simulink model "smm_with_grf_tilting_2d"  (R2014b)
settings: Solver=FixedStepDiscrete  StartTime=0.0  StopTime=inf  FixedStep=sample_time  RelTol=1e-3
undefined symbols (not defined in the file or in its folder): A_kalman_fourbar_gear, A_kalman_transverse, A_kalman_vertical, A_lpf_dtau, A_lpf_leg_spring, alpha_apex, B1_lpf_dtau, B1_lpf_leg_spring, B2_lpf_dtau, B2_lpf_leg_spring, B_kalman_fourbar_gear, B_kalman_transverse, B_kalman_vertical, b_virtual, boom_mount_angle, c_energy, C_kalman_fourbar_gear, C_kalman_transverse, C_kalman_vertical, com_leg_motor, com_torso, contact_threshold, control_start_time, d_vertical_boom_com_offset, d_vertical_com, d_y_com, desired_com_apex_height, desired_com_forward_velocity, desired_torso_angle, Discrete, fcut_contact, g, h_boom, HIP_MTR_MAX_CONT_TORQUE, i_robot, initial_dx_estimate, initial_dy_estimate, initial_dz_estimate, initial_z_estimate, j_leg, j_motor, j_rotor, j_segments, k0_virtual, k_placement, k_sea, kalman_load_to_deflect_transmission, kalman_stance_slip_threshold, kd_lateral, kd_motor, kd_torso, kp_lateral, kp_motor, kp_torso, l0_leg, l0_virtual, l_boom_projected, l_retract_delta, l_retract_swing_max, l_retract_swing_min ... (+59)
libraries: simulink x25, ctrlSharedLib x7, simulink_extras x1
(part 3 of 4)

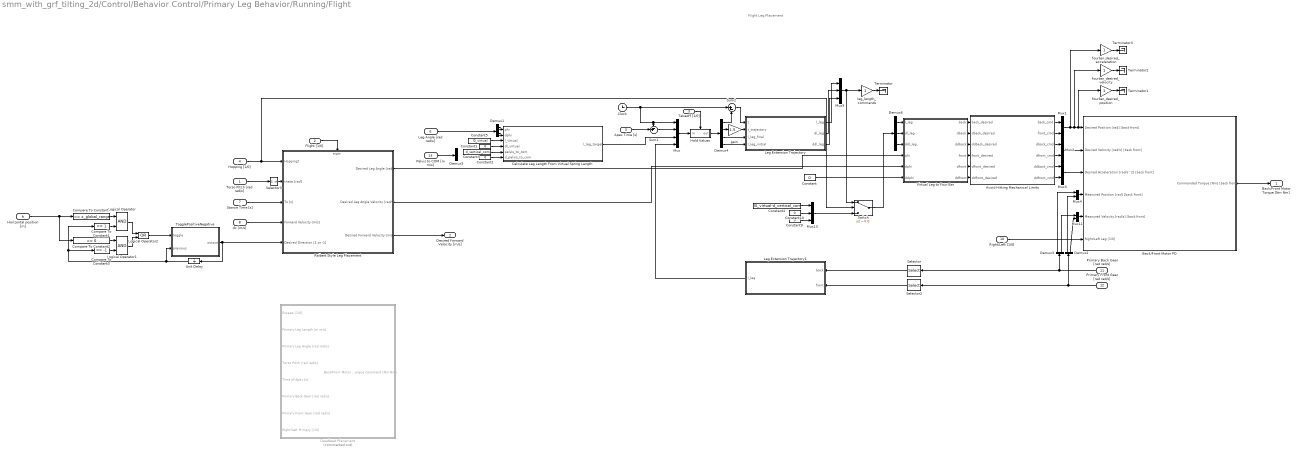
== system smm_with_grf_tilting_2d/Control/Behavior Control/Primary Leg Behavior/Running/Flight ==
  note: Flight
      | Leg Placement
  Torso Pitch [rad rad/s] : Inport
  Flight [1/0] : Inport  Port=2
  Takeoff [1/0] : Inport  Port=3
  Hopping [1/0] : Inport  Port=4
  Apex Time [s] : Inport  Port=5
  Leg Angle [rad rad/s] : Inport  Port=6
  Stance Time [s] : Inport  Port=7
  dx [m/s] : Inport  Port=8
  Horizontal position [m] : Inport  Port=9
  Right/Left [1/0] : Inport  Port=10
  Primary Back Gear [rad rad/s] : Inport  Port=11
  Primary Front Gear [rad rad/s] : Inport  Port=12
  Pelvis to COM [m m/s] : Inport  Port=13
  Avoid Hitting Mechanical Limits : MATLAB Function  TreatAsAtomicUnit=on
  Back/Front Motor PD : Subsystem
  Calculate Leg Length From Virtual Spring Length : MATLAB Function  TreatAsAtomicUnit=on
  Clock : Clock
  Compare To Constant : simulink/Logic and Bit Operations/Compare To Constant  relop=>=  const=x_global_range  OutDataTypeStr=boolean
  Compare To Constant1 : simulink/Logic and Bit Operations/Compare To Constant  relop===  const=1  OutDataTypeStr=boolean
  Compare To Constant2 : simulink/Logic and Bit Operations/Compare To Constant  relop=<=  const=0  OutDataTypeStr=boolean
  Compare To Constant3 : simulink/Logic and Bit Operations/Compare To Constant  relop===  const=-1  OutDataTypeStr=boolean
  Constant{,1..2,9..10} (5 alike) : Constant  Value=0
  Constant3 : Constant  Value=d_vertical_com
  Constant4 : Constant  Value=l0_virtual-d_vertical_com
  Constant5 : Constant  Value=l0_virtual
  Deadbeat Placement : Subsystem  Commented=on
  Demux{1..3,5} (4 alike) : Demux  Outputs=2
  Demux4 : Demux
  Demux6 : Demux  Outputs=3
  Hold Values : Subsystem
  Leg Extension Trajectory : MATLAB Function  TreatAsAtomicUnit=on
  Leg Extension Trajectory1 : MATLAB Function  TreatAsAtomicUnit=on
  Logical Operator : Logic  AllPortsSameDT=off  OutDataTypeStr=boolean
  Logical Operator1 : Logic  AllPortsSameDT=off  OutDataTypeStr=boolean
  Logical Operator2 : Logic  Operator=OR  AllPortsSameDT=off  OutDataTypeStr=boolean
  Mux : Mux
  Mux{1..4,11} (5 alike) : Mux  Inputs=2
  Mux13 : Mux  Inputs=3
  Mux5 : Mux  Inputs=3
  Raibert Style Leg Placement : Subsystem
  Selector : Selector  InputPortWidth=2  Indices=[1]
  Selector2 : Selector  InputPortWidth=2  Indices=[1]
  Selector3 : Selector  InputPortWidth=2  Indices=[1]
  Sum1 : Sum  Inputs=-+|
  Sum2 : Sum  Inputs=|+-
  Switch : Switch  Criteria=u2 ~= 0
  Terminator{,1..3} (4 alike) : Terminator
  TogglePositiveNegative : MATLAB Function  TreatAsAtomicUnit=on
      settings: MinAlgLoopOccurrences=on
  Unit Delay : UnitDelay  InitialCondition=1  SampleTime=sample_time
  Virtual Leg to Four Bar : MATLAB Function  TreatAsAtomicUnit=on
  fourbar_desired_acceleration : Gain
  fourbar_desired_position : Gain
  fourbar_desired_velocity : Gain
  gain : Gain  Gain=1.5
  leg_length_commands : Gain
  Back/Front Motor Torque [Nm Nm] : Outport
  Desired Forward Velocity [m/s] : Outport  Port=2
  wires:
  Hopping [1/0]/1 -> Switch/2, Raibert Style Leg Placement/1(Hopping?)
  Flight [1/0]/1 -> Raibert Style Leg Placement/Enable
  Selector3/1 -> Raibert Style Leg Placement/2(theta [rad])
  dx [m/s]/1 -> Raibert Style Leg Placement/4(Forward Velocity [m/s])
  Stance Time [s]/1 -> Raibert Style Leg Placement/3(Ts [s])
  Virtual Leg to Four Bar/1(back) -> Avoid Hitting Mechanical Limits/1(back_desired)
  Virtual Leg to Four Bar/2(dback) -> Avoid Hitting Mechanical Limits/2(dback_desired)
  Virtual Leg to Four Bar/3(ddback) -> Avoid Hitting Mechanical Limits/3(ddback_desired)
  Virtual Leg to Four Bar/4(front) -> Avoid Hitting Mechanical Limits/4(front_desired)
  Virtual Leg to Four Bar/5(dfront) -> Avoid Hitting Mechanical Limits/5(dfront_desired)
  Virtual Leg to Four Bar/6(ddfront) -> Avoid Hitting Mechanical Limits/6(ddfront_desired)
  Mux11/1 -> Back/Front Motor PD/5(Measured Velocity [rad/s] [back front])
  Demux2/2 -> Mux11/2
  Mux4/1 -> Back/Front Motor PD/4(Measured Position [rad] [back front])
  Mux1/1 -> fourbar_desired_acceleration/1, fourbar_desired_velocity/1, fourbar_desired_position/1, Back/Front Motor PD/1(Desired Position [rad] [back front])
  Demux3/2 -> Mux11/1
  Demux3/1 -> Mux4/1
  Avoid Hitting Mechanical Limits/2(front_cmd) -> Mux1/2
  Avoid Hitting Mechanical Limits/1(back_cmd) -> Mux1/1
  Demux2/1 -> Mux4/2
  Avoid Hitting Mechanical Limits/3(dback_cmd) -> Mux2/1
  Avoid Hitting Mechanical Limits/4(dfront_cmd) -> Mux2/2
  Avoid Hitting Mechanical Limits/5(ddback_cmd) -> Mux3/1
  Avoid Hitting Mechanical Limits/6(ddfront_cmd) -> Mux3/2
  Mux2/1 -> Back/Front Motor PD/2(Desired Velocity [rad/s] [back front])
  Mux3/1 -> Back/Front Motor PD/3(Desired Acceleration [rad/s^2] [back front])
  Back/Front Motor PD/1(Commanded Torque [Nm] [back front]) -> Back/Front Motor Torque [Nm Nm]/1
  Primary Back Gear [rad rad/s]/1 -> Demux3/1, Selector/1
  Primary Front Gear [rad rad/s]/1 -> Demux2/1, Selector2/1
  Constant/1 -> Virtual Leg to Four Bar/6(ddphi)
  Raibert Style Leg Placement/1(Desired Leg Angle [rad]) -> Virtual Leg to Four Bar/4(phi)
  Raibert Style Leg Placement/2(Desired Leg Angle Velocity [rad/s]) -> Virtual Leg to Four Bar/5(dphi)
  Constant5/1 -> Calculate Leg Length From Virtual Spring Length/3(l_virtual)
  Constant1/1 -> Calculate Leg Length From Virtual Spring Length/4(dl_virtual)
  Demux1/1 -> Calculate Leg Length From Virtual Spring Length/1(phi)
  Demux1/2 -> Calculate Leg Length From Virtual Spring Length/2(dphi)
  Apex Time [s]/1 -> Sum1/2
  Clock/1 -> Sum1/1, Mux/1, Sum2/1
  Sum2/1 -> Leg Extension Trajectory/1(t)
  Mux5/1 -> Switch/1, leg_length_commands/1
  leg_length_commands/1 -> Terminator/1
  Demux4/2 -> gain/1
  Sum1/1 -> Mux/2
  Calculate Leg Length From Virtual Spring Length/1(l_leg_target) -> Mux/3
  Demux4/4 -> Leg Extension Trajectory/4(l_leg_initial)
  Demux4/3 -> Leg Extension Trajectory/3(l_leg_final)
  Demux4/1 -> Sum2/2
  Selector/1 -> Leg Extension Trajectory1/1(back)
  Selector2/1 -> Leg Extension Trajectory1/2(front)
  Right/Left [1/0]/1 -> Back/Front Motor PD/6(Right/Left Leg [1/0])
  Hold Values/1(out) -> Demux4/1
  Mux/1 -> Hold Values/1(in)
  gain/1 -> Leg Extension Trajectory/2(t_trajectory)
  Takeoff [1/0]/1 -> Hold Values/Trigger
  Leg Extension Trajectory1/1(l_leg) -> Mux/4
  Leg Angle [rad rad/s]/1 -> Demux1/1
  TogglePositiveNegative/1(output) -> Raibert Style Leg Placement/5(Desired Direction [1 or -1]), Unit Delay/1
  Torso Pitch [rad rad/s]/1 -> Selector3/1
  fourbar_desired_position/1 -> Terminator1/1
  fourbar_desired_velocity/1 -> Terminator2/1
  fourbar_desired_acceleration/1 -> Terminator3/1
  Pelvis to COM [m m/s]/1 -> Demux5/1
  Constant2/1 -> Calculate Leg Length From Virtual Spring Length/6(d_pelvis_to_com)
  Constant3/1 -> Calculate Leg Length From Virtual Spring Length/5(pelvis_to_com)
  Horizontal position [m]/1 -> Compare To Constant2/1, Compare To Constant/1
  Unit Delay/1 -> TogglePositiveNegative/2(previous), Compare To Constant3/1, Compare To Constant1/1
  Compare To Constant/1 -> Logical Operator/1
  Compare To Constant1/1 -> Logical Operator/2
  Compare To Constant2/1 -> Logical Operator1/1
  Compare To Constant3/1 -> Logical Operator1/2
  Logical Operator1/1 -> Logical Operator2/2
  Logical Operator2/1 -> TogglePositiveNegative/1(toggle)
  Logical Operator/1 -> Logical Operator2/1
  Raibert Style Leg Placement/3(Desired Forward Velocity [m/s]) -> Desired Forward Velocity [m/s]/1
  Leg Extension Trajectory/1(l_leg) -> Mux5/1
  Leg Extension Trajectory/2(dl_leg) -> Mux5/2
  Leg Extension Trajectory/3(ddl_leg) -> Mux5/3
  Constant4/1 -> Mux13/1
  Constant9/1 -> Mux13/3
  Constant10/1 -> Mux13/2
  Mux13/1 -> Switch/3
  Demux6/2 -> Virtual Leg to Four Bar/2(dl_leg)
  Demux6/1 -> Virtual Leg to Four Bar/1(l_leg)
  Demux6/3 -> Virtual Leg to Four Bar/3(ddl_leg)
  Switch/1 -> Demux6/1

== system smm_with_grf_tilting_2d/Control/Behavior Control/Primary Leg Behavior/Running/Stance ==
  note: Stance
      | Virtual Spring Force / Posture Control
  System Energy [J] : Inport
  Leg Length [m m/s] : Inport  Port=2
  Torso Pitch [rad rad/s] : Inport  Port=3
  Primary w [m] : Inport  Port=4
  Virtual Spring Length [m m/s] : Inport  Port=5
  Primary Leg Force [N] : Inport  Port=6
  Stance [1/0] : Inport  Port=7
  Leg Angle [rad rad/s] : Inport  Port=8
  Hopping [1/0] : Inport  Port=9
  Right/Left Primary [1/0] : Inport  Port=10
  Desired Forward Velocity [m/s] : Inport  Port=11
  Calculate Spring Rest Length : Subsystem
  Inverse Dynamics Virtual Spring : Subsystem
  Nonlinear Spring Stiffness : Subsystem
  Selector1 : Selector  InputPortWidth=2  Indices=[2]
  Selector4 : Selector  InputPortWidth=2  Indices=[1]
  Terminator1 : Terminator
  Terminator2 : Terminator
  Virtual Spring Stance Rest Length : Gain
  Virtual Spring Stiffness : Gain
  Leg Force Command (stance) [N] : Outport
  Leg Torque Command (stance) [Nm] : Outport  Port=2
  wires:
  Inverse Dynamics Virtual Spring/2(Leg Torque [Nm]) -> Leg Torque Command (stance) [Nm]/1
  Torso Pitch [rad rad/s]/1 -> Inverse Dynamics Virtual Spring/4(Torso Pitch [rad rad/s])
  System Energy [J]/1 -> Nonlinear Spring Stiffness/2(System Energy [J])
  Primary Leg Force [N]/1 -> Calculate Spring Rest Length/3(Measured Leg Force)
  Selector4/1 -> Calculate Spring Rest Length/2(Virtual Spring Length [m])
  Calculate Spring Rest Length/1(Rest Length [m]) -> Virtual Spring Stance Rest Length/1, Inverse Dynamics Virtual Spring/7(Spring Rest Length [m])
  Virtual Spring Stance Rest Length/1 -> Terminator2/1
  Virtual Spring Stiffness/1 -> Terminator1/1
  Primary w [m]/1 -> Inverse Dynamics Virtual Spring/5(Primary w [m])
  Virtual Spring Length [m m/s]/1 -> Selector4/1, Inverse Dynamics Virtual Spring/6(Virtual Spring Length [m m/s]), Selector1/1
  Leg Length [m m/s]/1 -> Inverse Dynamics Virtual Spring/2(Leg Length [m m/s])
  Selector1/1 -> Nonlinear Spring Stiffness/1(Virtual Spring Velocity [m/s])
  Nonlinear Spring Stiffness/1(Virtual Spring Stiffness [N/m]) -> Calculate Spring Rest Length/1(Spring Constant), Virtual Spring Stiffness/1, Inverse Dynamics Virtual Spring/1(k_virtual [N/m])
  Stance [1/0]/1 -> Calculate Spring Rest Length/4(Contact [1/0])
  Leg Angle [rad rad/s]/1 -> Inverse Dynamics Virtual Spring/3(Leg Angle [rad rad/s])
  Hopping [1/0]/1 -> Inverse Dynamics Virtual Spring/8(Hopping [1/0])
  Right/Left Primary [1/0]/1 -> Inverse Dynamics Virtual Spring/9(Right/Left [1/0])
  Desired Forward Velocity [m/s]/1 -> Nonlinear Spring Stiffness/3(Desired Forward Velocity [m/s])
  Inverse Dynamics Virtual Spring/1(Leg Force [N]) -> Leg Force Command (stance) [N]/1

== system smm_with_grf_tilting_2d/Control/Behavior Control/Secondary Leg Behavior/Back//Front Motor PD/Friction Compensation ==
  Right/Left [1/0] : Inport
  Commanded Velocity [rad/s] [back front] : Inport  Port=2
  Product : Product
  Sign : Signum
  Sum1 : Sum
  Switch : Switch  Criteria=u2 ~= 0
  Switch1 : Switch  Criteria=u2 ~= 0
  coulomb_friction_left : Constant  Value=sea_coulomb_friction(3:4)
  coulomb_friction_right : Constant  Value=sea_coulomb_friction(1:2)
  offset_friction_left : Constant  Value=sea_offset_friction(3:4)
  offset_friction_right : Constant  Value=sea_offset_friction(1:2)
  Friction Compensation [Nm] : Outport
  wires:
  Commanded Velocity [rad/s] [back front]/1 -> Sign/1
  Switch/1 -> Sum1/2
  Sum1/1 -> Friction Compensation [Nm]/1
  Product/1 -> Sum1/1
  Right/Left [1/0]/1 -> Switch1/2, Switch/2
  offset_friction_right/1 -> Switch/1
  offset_friction_left/1 -> Switch/3
  coulomb_friction_right/1 -> Switch1/1
  coulomb_friction_left/1 -> Switch1/3
  Switch1/1 -> Product/2
  Sign/1 -> Product/1

== system smm_with_grf_tilting_2d/Control/Behavior Control/Primary Leg Behavior/Running/Flight/Back//Front Motor PD ==
  Desired Position [rad] [back front] : Inport
  Desired Velocity [rad/s] [back front] : Inport  Port=2
  Desired Acceleration [rad/s^2] [back front] : Inport  Port=3
  Measured Position [rad] [back front] : Inport  Port=4
  Measured Velocity [rad/s] [back front] : Inport  Port=5
  Right/Left Leg [1/0] : Inport  Port=6
  Friction Compensation : Subsystem
  Product : Product
  Sum1 : Sum  Inputs=|++
  Sum2 : Sum  Inputs=|++
  Sum7 : Sum  Inputs=|+-
  Sum8 : Sum  Inputs=|+-
  Sum9 : Sum
  kd : Gain  Gain=kd_motor
  kp : Gain  Gain=kp_motor
  reflected inertia : Constant  Value=j_motor
  Commanded Torque [Nm] [back front] : Outport
  wires:
  kp/1 -> Sum9/1
  Sum7/1 -> kp/1
  Measured Position [rad] [back front]/1 -> Sum7/2
  Sum9/1 -> Sum1/1
  Sum8/1 -> kd/1
  Desired Position [rad] [back front]/1 -> Sum7/1
  kd/1 -> Sum9/2
  Measured Velocity [rad/s] [back front]/1 -> Sum8/2
  Sum1/1 -> Sum2/1
  Desired Acceleration [rad/s^2] [back front]/1 -> Product/1
  Product/1 -> Sum1/2
  Right/Left Leg [1/0]/1 -> Friction Compensation/1(Right/Left [1/0])
  Sum2/1 -> Commanded Torque [Nm] [back front]/1
  Desired Velocity [rad/s] [back front]/1 -> Friction Compensation/2(Commanded Velocity [rad/s] [back front]), Sum8/1
  reflected inertia/1 -> Product/2
  Friction Compensation/1(Friction Compensation [Nm]) -> Sum2/2

== system smm_with_grf_tilting_2d/Control/Behavior Control/Primary Leg Behavior/Running/Flight/Deadbeat Placement ==
  note: Convert to
      | four-bar angles
  note: Primary Swing Behavior
  note: Position control the
      | individual four bar segments
  note: Generate a virtual
      | leg trajectory
  Escape [1/0] : Inport
  Primary Leg Length [m m/s] : Inport  Port=2
  Primary Leg Angle [rad rad/s] : Inport  Port=3
  Torso Pitch [rad rad/s] : Inport  Port=4
  Time of Apex [s] : Inport  Port=5
  Primary Back Gear [rad rad/s] : Inport  Port=6
  Primary Front Gear [rad rad/s] : Inport  Port=7
  Right/Left Primary [1/0] : Inport  Port=8
  Avoid Hitting Mechanical Limits1 : MATLAB Function  TreatAsAtomicUnit=on
  Back/Front Motor PD : Subsystem
  Demux1 : Demux  Outputs=3
  Demux2 : Demux  Outputs=3
  Demux3 : Demux  Outputs=2
  Demux5 : Demux  Outputs=2
  Leg Trajectory Generator (Level Ground) : Subsystem  Commented=on
  Leg Trajectory Generator (Normal) : Subsystem
  LegAngleTarget : Gain
  LegLengthTarget : Gain
  Mux{1..3,7..8} (5 alike) : Mux  Inputs=2
  Terminator1 : Terminator
  Terminator5 : Terminator
  Virtual Leg to Four Bar : MATLAB Function  TreatAsAtomicUnit=on
  Back/Front Motor Torque Command [Nm Nm] : Outport
  wires:
  LegAngleTarget/1 -> Terminator1/1
  Leg Trajectory Generator (Normal)/1(Leg Length Target [m m/s m/s^2]) -> LegLengthTarget/1, Demux2/1
  LegLengthTarget/1 -> Terminator5/1
  Mux3/1 -> Back/Front Motor PD/3(Desired Acceleration [rad/s^2] [back front])
  Mux2/1 -> Back/Front Motor PD/2(Desired Velocity [rad/s] [back front])
  Avoid Hitting Mechanical Limits1/6(ddfront_cmd) -> Mux3/2
  Avoid Hitting Mechanical Limits1/5(ddback_cmd) -> Mux3/1
  Avoid Hitting Mechanical Limits1/4(dfront_cmd) -> Mux2/2
  Avoid Hitting Mechanical Limits1/3(dback_cmd) -> Mux2/1
  Primary Back Gear [rad rad/s]/1 -> Demux3/1
  Primary Front Gear [rad rad/s]/1 -> Demux5/1
  Demux2/1 -> Virtual Leg to Four Bar/1(l_leg)
  Demux1/2 -> Virtual Leg to Four Bar/5(dphi)
  Demux1/1 -> Virtual Leg to Four Bar/4(phi)
  Demux2/2 -> Virtual Leg to Four Bar/2(dl_leg)
  Demux1/3 -> Virtual Leg to Four Bar/6(ddphi)
  Demux2/3 -> Virtual Leg to Four Bar/3(ddl_leg)
  Back/Front Motor PD/1(Commanded Torque [Nm] [back front]) -> Back/Front Motor Torque Command [Nm Nm]/1
  Demux5/1 -> Mux7/2
  Avoid Hitting Mechanical Limits1/1(back_cmd) -> Mux1/1
  Virtual Leg to Four Bar/1(back) -> Avoid Hitting Mechanical Limits1/1(back_desired)
  Avoid Hitting Mechanical Limits1/2(front_cmd) -> Mux1/2
  Virtual Leg to Four Bar/3(ddback) -> Avoid Hitting Mechanical Limits1/3(ddback_desired)
  Virtual Leg to Four Bar/6(ddfront) -> Avoid Hitting Mechanical Limits1/6(ddfront_desired)
  Virtual Leg to Four Bar/4(front) -> Avoid Hitting Mechanical Limits1/4(front_desired)
  Virtual Leg to Four Bar/2(dback) -> Avoid Hitting Mechanical Limits1/2(dback_desired)
  Demux3/1 -> Mux7/1
  Demux3/2 -> Mux8/1
  Torso Pitch [rad rad/s]/1 -> Leg Trajectory Generator (Normal)/3(Torso Pitch [rad rad/s])
  Right/Left Primary [1/0]/1 -> Back/Front Motor PD/6(Right/Left Leg [1/0])
  Primary Leg Angle [rad rad/s]/1 -> Leg Trajectory Generator (Normal)/2(Leg Angle [rad rad/s])
  Primary Leg Length [m m/s]/1 -> Leg Trajectory Generator (Normal)/1(Leg Length [m m/s])
  Mux1/1 -> Back/Front Motor PD/1(Desired Position [rad] [back front])
  Mux7/1 -> Back/Front Motor PD/4(Measured Position [rad] [back front])
  Virtual Leg to Four Bar/5(dfront) -> Avoid Hitting Mechanical Limits1/5(dfront_desired)
  Time of Apex [s]/1 -> Leg Trajectory Generator (Normal)/4(Apex Time [s])
  Demux5/2 -> Mux8/2
  Mux8/1 -> Back/Front Motor PD/5(Measured Velocity [rad/s] [back front])
  Escape [1/0]/1 -> Leg Trajectory Generator (Normal)/5(Escape [1/0])
  Leg Trajectory Generator (Normal)/2(Leg Angle Target [rad rad/s rad/s^2]) -> LegAngleTarget/1, Demux1/1

== system smm_with_grf_tilting_2d/Control/Behavior Control/Primary Leg Behavior/Running/Flight/Hold Values ==
  in : Inport
  Trigger : TriggerPort  ShowOutputPort=on  PortDimensions=1
  Subsystem : Subsystem
  out : Outport
  wires:
  in/1 -> Subsystem/1(in)
  Subsystem/1(out) -> out/1
  Trigger/1 -> Subsystem/Enable

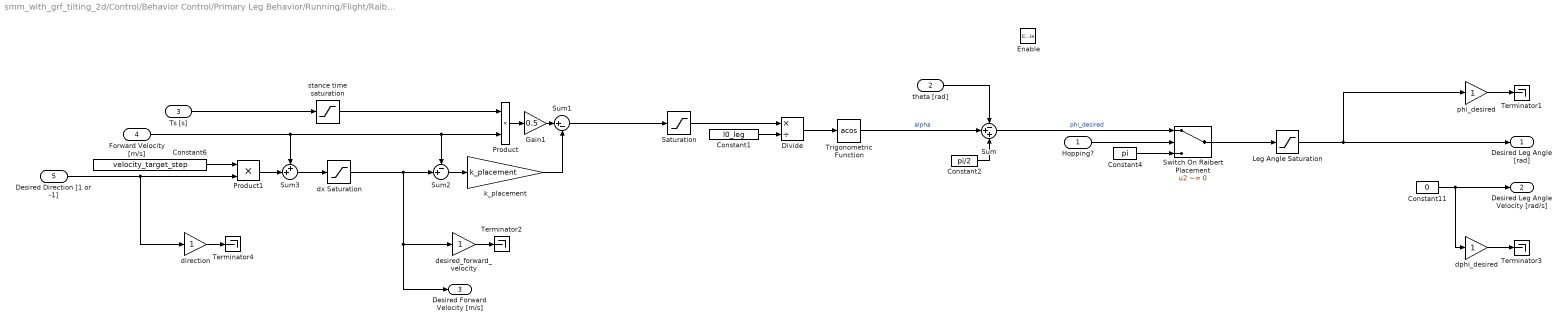
== system smm_with_grf_tilting_2d/Control/Behavior Control/Primary Leg Behavior/Running/Flight/Raibert Style Leg Placement ==
  Hopping? : Inport
  theta [rad] : Inport  Port=2
  Ts [s] : Inport  Port=3
  Forward Velocity [m/s] : Inport  Port=4
  Desired Direction [1 or -1] : Inport  Port=5
  Enable : EnablePort
  Constant1 : Constant  Value=l0_leg
  Constant11 : Constant  Value=0
  Constant2 : Constant  Value=pi/2
  Constant4 : Constant  Value=pi
  Constant6 : Constant  Value=velocity_target_step
  Divide : Product  Inputs=*/
  Gain1 : Gain  Gain=0.5
  Leg Angle Saturation : Saturate  UpperLimit=max_leg_angle  LowerLimit=min_leg_angle
      settings: AttributesFormatString=Hi: %<UpperLimit>\nLo: %<LowerLimit>
  Product : Product
  Product1 : Product
  Saturation : Saturate  UpperLimit=x_limit  LowerLimit=-x_limit
      settings: AttributesFormatString=Hi: %<UpperLimit>\nLo: %<LowerLimit>
  Sum : Sum  Inputs=-++
  Sum1 : Sum  Inputs=|+-
  Sum2 : Sum  Inputs=-+|
  Sum3 : Sum  Inputs=++|
  Switch On Raibert Placement : Switch  Criteria=u2 ~= 0
  Terminator{1..4} (4 alike) : Terminator
  Trigonometric Function : Trigonometry  Operator=acos
  desired_forward_velocity : Gain
  direction : Gain
  dphi_desired : Gain
  dx Saturation : Saturate  UpperLimit=desired_com_forward_velocity  LowerLimit=-desired_com_forward_velocity
      settings: AttributesFormatString=Hi: %<UpperLimit>\nLo: %<LowerLimit>
  k_placement : Gain  Gain=k_placement
  phi_desired : Gain
  stance time saturation : Saturate  UpperLimit=1  LowerLimit=0
      settings: AttributesFormatString=Hi: %<UpperLimit>\nLo: %<LowerLimit>
  Desired Leg Angle [rad] : Outport  OutputWhenDisabled=reset  InitialOutput=[0]
  Desired Leg Angle Velocity [rad/s] : Outport  Port=2  OutputWhenDisabled=reset  InitialOutput=[0]
  Desired Forward Velocity [m/s] : Outport  Port=3  InitialOutput=[0]
  wires:
  Sum2/1 -> k_placement/1
  Ts [s]/1 -> stance time saturation/1
  Product/1 -> Gain1/1
  Gain1/1 -> Sum1/1
  Saturation/1 -> Divide/1
  Constant1/1 -> Divide/2
  Divide/1 -> Trigonometric Function/1
  Trigonometric Function/1 -> Sum/2  "alpha"
  Constant2/1 -> Sum/3
  theta [rad]/1 -> Sum/1
  Sum/1 -> Switch On Raibert Placement/1  "phi_desired"
  Sum1/1 -> Saturation/1
  Constant4/1 -> Switch On Raibert Placement/3
  Hopping?/1 -> Switch On Raibert Placement/2
  Leg Angle Saturation/1 -> Desired Leg Angle [rad]/1, phi_desired/1
  Switch On Raibert Placement/1 -> Leg Angle Saturation/1
  Sum3/1 -> dx Saturation/1
  Forward Velocity [m/s]/1 -> Sum3/1, Sum2/1, Product/2
  Product1/1 -> Sum3/2
  stance time saturation/1 -> Product/1
  k_placement/1 -> Sum1/2
  Constant6/1 -> Product1/1
  phi_desired/1 -> Terminator1/1
  dx Saturation/1 -> Desired Forward Velocity [m/s]/1, desired_forward_velocity/1, Sum2/2
  desired_forward_velocity/1 -> Terminator2/1
  Constant11/1 -> dphi_desired/1, Desired Leg Angle Velocity [rad/s]/1
  dphi_desired/1 -> Terminator3/1
  Desired Direction [1 or -1]/1 -> direction/1, Product1/2
  direction/1 -> Terminator4/1

== system smm_with_grf_tilting_2d/Control/Behavior Control/Primary Leg Behavior/Running/Stance/Calculate Spring Rest Length ==
  Spring Constant : Inport
  Virtual Spring Length [m] : Inport  Port=2
  Measured Leg Force : Inport  Port=3
  Contact [1/0] : Inport  Port=4
  Constant5 : Constant  Value=l0_virtual
  Divide : Product  Inputs=*/
  Hold Initial : Subsystem
  Saturation : Saturate  UpperLimit=inf  LowerLimit=0
  Sum3 : Sum  Inputs=++|
  Rest Length [m] : Outport
  wires:
  Divide/1 -> Sum3/2
  Virtual Spring Length [m]/1 -> Sum3/1
  Measured Leg Force/1 -> Saturation/1
  Sum3/1 -> Hold Initial/1(in)
  Constant5/1 -> Rest Length [m]/1
  Saturation/1 -> Divide/1
  Contact [1/0]/1 -> Hold Initial/Trigger
  Spring Constant/1 -> Divide/2

== system smm_with_grf_tilting_2d/Control/Behavior Control/Primary Leg Behavior/Running/Stance/Inverse Dynamics Virtual Spring ==
  k_virtual [N/m] : Inport
  Leg Length [m m/s] : Inport  Port=2
  Leg Angle [rad rad/s] : Inport  Port=3
  Torso Pitch [rad rad/s] : Inport  Port=4
  Primary w [m] : Inport  Port=5
  Virtual Spring Length [m m/s] : Inport  Port=6
  Spring Rest Length [m] : Inport  Port=7
  Hopping [1/0] : Inport  Port=8
  Right/Left [1/0] : Inport  Port=9
  Constant1 : Constant  Value=b_virtual
  Constant2 : Constant  Value=0
  Constant3 : Constant  Value=desired_torso_angle
  Constant4 : Constant  Value=0
  Demux5 : Demux  Outputs=2
  GRF_angle : Gain
  GRFx_target : Gain
  GRFy_target : Gain
  Leg Force-Torque Distribution : Subsystem
  Spring Torques : Selector  InputPortWidth=7  Indices=[6 7]
  Switch : Switch  Criteria=u2 ~= 0
  Terminator : Terminator
  Terminator1 : Terminator
  Terminator2 : Terminator
  target_GRF_inverse_dynamics : MATLAB Function  TreatAsAtomicUnit=on
  Leg Force [N] : Outport
  Leg Torque [Nm] : Outport  Port=2
  wires:
  Leg Force-Torque Distribution/1(Leg Force [N]) -> Leg Force [N]/1
  GRF_angle/1 -> Terminator2/1
  GRFy_target/1 -> Terminator1/1
  GRFx_target/1 -> Terminator/1
  Leg Angle [rad rad/s]/1 -> target_GRF_inverse_dynamics/6(phi)
  Torso Pitch [rad rad/s]/1 -> target_GRF_inverse_dynamics/5(theta)
  target_GRF_inverse_dynamics/4(GRF_angle) -> GRF_angle/1
  target_GRF_inverse_dynamics/3(GRFy) -> GRFy_target/1
  target_GRF_inverse_dynamics/2(GRFx) -> GRFx_target/1
  Leg Force-Torque Distribution/2(Leg Torque [Nm]) -> Leg Torque [Nm]/1
  Primary w [m]/1 -> target_GRF_inverse_dynamics/8(w), Leg Force-Torque Distribution/3(w [m])
  Spring Torques/1 -> Demux5/1
  Demux5/1 -> Leg Force-Torque Distribution/1(Front Spring Torque [Nm])
  Demux5/2 -> Leg Force-Torque Distribution/2(Back Spring Torque [Nm])
  target_GRF_inverse_dynamics/1(z) -> Spring Torques/1
  Constant2/1 -> target_GRF_inverse_dynamics/10(tau_rotor_b), target_GRF_inverse_dynamics/9(tau_rotor_f)
  Leg Length [m m/s]/1 -> target_GRF_inverse_dynamics/7(l_leg)
  k_virtual [N/m]/1 -> target_GRF_inverse_dynamics/2(k_virtual)
  Virtual Spring Length [m m/s]/1 -> target_GRF_inverse_dynamics/4(l_virtual)
  Spring Rest Length [m]/1 -> target_GRF_inverse_dynamics/11(l_virtual_rest)
  Switch/1 -> target_GRF_inverse_dynamics/12(desired_torso_angle)
  Constant1/1 -> target_GRF_inverse_dynamics/3(b_virtual)
  Hopping [1/0]/1 -> Switch/2
  Constant3/1 -> Switch/1
  Constant4/1 -> Switch/3
  Right/Left [1/0]/1 -> target_GRF_inverse_dynamics/1(right_left)

== system smm_with_grf_tilting_2d/Control/Behavior Control/Primary Leg Behavior/Running/Stance/Nonlinear Spring Stiffness ==
  Virtual Spring Velocity [m/s] : Inport
  System Energy [J] : Inport  Port=2
  Desired Forward Velocity [m/s] : Inport  Port=3
  Math Function : Math  Operator=square  SaturateOnIntegerOverflow=on
  Product : Product  Inputs=3
  Product1 : Product
  Saturation : Saturate  UpperLimit=max_k_virtual  LowerLimit=min_k_virtual  ZeroCross=off
  Sum : Sum  Inputs=+|+
  Sum1 : Sum  Inputs=+-|
  Sum2 : Sum  Inputs=|++
  Terminator1 : Terminator
  c_energy : Constant  Value=c_energy
  desired potential energy : Constant  Value=desired_com_apex_height*m_total_real*g
  desired_system_energy : Gain
  half mass : Constant  Value=0.5*m_total_real
  k0_virtual : Constant  Value=k0_virtual
  Virtual Spring Stiffness [N/m] : Outport
  wires:
  Virtual Spring Velocity [m/s]/1 -> Product/2
  c_energy/1 -> Product/3
  k0_virtual/1 -> Sum/1
  Saturation/1 -> Virtual Spring Stiffness [N/m]/1
  Sum/1 -> Saturation/1
  Product/1 -> Sum/2
  System Energy [J]/1 -> Sum1/2
  desired potential energy/1 -> Sum2/1
  half mass/1 -> Product1/1
  Desired Forward Velocity [m/s]/1 -> Math Function/1
  Product1/1 -> Sum2/2
  desired_system_energy/1 -> Terminator1/1
  Sum2/1 -> Sum1/1, desired_system_energy/1
  Math Function/1 -> Product1/2
  Sum1/1 -> Product/1

== system smm_with_grf_tilting_2d/Control/Behavior Control/Primary Leg Behavior/Running/Flight/Back//Front Motor PD/Friction Compensation ==
  Right/Left [1/0] : Inport
  Commanded Velocity [rad/s] [back front] : Inport  Port=2
  Product : Product
  Sign : Signum
  Sum1 : Sum
  Switch : Switch  Criteria=u2 ~= 0
  Switch1 : Switch  Criteria=u2 ~= 0
  coulomb_friction_left : Constant  Value=sea_coulomb_friction(3:4)
  coulomb_friction_right : Constant  Value=sea_coulomb_friction(1:2)
  offset_friction_left : Constant  Value=sea_offset_friction(3:4)
  offset_friction_right : Constant  Value=sea_offset_friction(1:2)
  Friction Compensation [Nm] : Outport
  wires:
  Commanded Velocity [rad/s] [back front]/1 -> Sign/1
  Switch/1 -> Sum1/2
  Sum1/1 -> Friction Compensation [Nm]/1
  Product/1 -> Sum1/1
  Right/Left [1/0]/1 -> Switch1/2, Switch/2
  offset_friction_right/1 -> Switch/1
  offset_friction_left/1 -> Switch/3
  coulomb_friction_right/1 -> Switch1/1
  coulomb_friction_left/1 -> Switch1/3
  Switch1/1 -> Product/2
  Sign/1 -> Product/1

== system smm_with_grf_tilting_2d/Control/Behavior Control/Primary Leg Behavior/Running/Flight/Deadbeat Placement/Back//Front Motor PD ==
  Desired Position [rad] [back front] : Inport
  Desired Velocity [rad/s] [back front] : Inport  Port=2
  Desired Acceleration [rad/s^2] [back front] : Inport  Port=3
  Measured Position [rad] [back front] : Inport  Port=4
  Measured Velocity [rad/s] [back front] : Inport  Port=5
  Right/Left Leg [1/0] : Inport  Port=6
  Friction Compensation : Subsystem
  Product : Product
  Sum1 : Sum  Inputs=|++
  Sum2 : Sum  Inputs=|++
  Sum7 : Sum  Inputs=|+-
  Sum8 : Sum  Inputs=|+-
  Sum9 : Sum
  Switch : Switch  Criteria=u2 ~= 0
  kd : Gain  Gain=kd_motor
  kp : Gain  Gain=kp_motor
  left_inertias : Constant  Value=j_segments(3:4)
  right_inertias : Constant  Value=j_segments(1:2)
  Commanded Torque [Nm] [back front] : Outport
  wires:
  kp/1 -> Sum9/1
  Sum7/1 -> kp/1
  Measured Position [rad] [back front]/1 -> Sum7/2
  Sum9/1 -> Sum1/1
  Sum8/1 -> kd/1
  Desired Position [rad] [back front]/1 -> Sum7/1
  kd/1 -> Sum9/2
  Measured Velocity [rad/s] [back front]/1 -> Sum8/2
  Sum1/1 -> Sum2/1
  Desired Acceleration [rad/s^2] [back front]/1 -> Product/1
  Product/1 -> Sum1/2
  Right/Left Leg [1/0]/1 -> Friction Compensation/1(Right/Left [1/0]), Switch/2
  right_inertias/1 -> Switch/1
  left_inertias/1 -> Switch/3
  Switch/1 -> Product/2
  Sum2/1 -> Commanded Torque [Nm] [back front]/1
  Friction Compensation/1(Friction Compensation [Nm]) -> Sum2/2
  Desired Velocity [rad/s] [back front]/1 -> Friction Compensation/2(Commanded Velocity [rad/s] [back front]), Sum8/1

== system smm_with_grf_tilting_2d/Control/Behavior Control/Primary Leg Behavior/Running/Flight/Deadbeat Placement/Leg Trajectory Generator (Level Ground) ==
  Leg Length [m m/s] : Inport
  Leg Angle [rad rad/s] : Inport  Port=2
  Torso Pitch [rad rad/s] : Inport  Port=3
  Apex Time [s] : Inport  Port=4
  Escape [1/0] : Inport  Port=5
  Alpha Target Law l0 = 1.037112 m k = 23000 N/m target height = 1.137112 m target speed = 0.5 m/s m = 60.4120 kg g = 5.9004 m/s^2 E = 412.882588 J : Subsystem
  Alpha Target to Leg Length and Leg Angle : MATLAB Function  TreatAsAtomicUnit=on
  AlphaRef : Gain
  Clock : Clock
  Compare To Constant : simulink/Logic and Bit Operations/Compare To Constant  relop=>  const=0  OutDataTypeStr=boolean  ZeroCross=off
  Demux : Demux  Outputs=6
  Demux1 : Demux  Outputs=2
  Demux2 : Demux  Outputs=2
  Demux3 : Demux  Outputs=2
  Detect Fall Nonpositive : simulink/Logic and Bit Operations/Detect Fall Nonpositive  vinit=0  InputProcessing=Inherited  OutDataTypeStr=boolean
  Gain : Gain  Gain=-1
  Mux1 : Mux  Inputs=6
  Mux2 : Mux  Inputs=3
  Mux3 : Mux  Inputs=3
  Mux4 : Mux  Inputs=6
  Retracted Leg Trajectory : MATLAB Function  TreatAsAtomicUnit=on
  Signal During Escape : Subsystem
  Sum1 : Sum  Inputs=|+-
  Switch : Switch  Criteria=u2 ~= 0
  Terminator5 : Terminator
  Leg Length Target [m m/s m/s^2] : Outport
  Leg Angle Target [rad rad/s rad/s^2] : Outport  Port=2
  wires:
  Gain/1 -> Alpha Target Law l0 = 1.037112 m k = 23000 N/m target height = 1.137112 m target speed = 0.5 m/s m = 60.4120 kg g = 5.9004 m/s^2 E = 412.882588 J/1(tFall [s])
  Signal During Escape/1(time to apex [s]) -> Gain/1
  Leg Length [m m/s]/1 -> Demux2/1
  Leg Angle [rad rad/s]/1 -> Demux3/1
  Demux3/2 -> Retracted Leg Trajectory/11(dphi_measured)
  Demux3/1 -> Retracted Leg Trajectory/10(phi_measured)
  Demux2/2 -> Retracted Leg Trajectory/9(dl_measured)
  Demux2/1 -> Retracted Leg Trajectory/8(l_measured)
  Retracted Leg Trajectory/6(ddphi) -> Mux1/6
  Retracted Leg Trajectory/3(ddl) -> Mux1/3
  Mux4/1 -> Switch/1
  Demux1/2 -> Alpha Target to Leg Length and Leg Angle/5(dtheta)
  Demux1/1 -> Alpha Target to Leg Length and Leg Angle/4(theta)
  Demux/1 -> Mux2/1
  Demux/2 -> Mux2/2
  Demux/3 -> Mux2/3
  Demux/4 -> Mux3/1
  Demux/5 -> Mux3/2
  Demux/6 -> Mux3/3
  Mux3/1 -> Leg Angle Target [rad rad/s rad/s^2]/1
  Mux2/1 -> Leg Length Target [m m/s m/s^2]/1
  Switch/1 -> Demux/1
  Alpha Target to Leg Length and Leg Angle/1(l) -> Mux4/1, Retracted Leg Trajectory/4(l_apex)
  Alpha Target to Leg Length and Leg Angle/2(dl) -> Mux4/2, Retracted Leg Trajectory/5(dl_apex)
  Alpha Target to Leg Length and Leg Angle/6(ddphi) -> Mux4/6
  Alpha Target to Leg Length and Leg Angle/5(dphi) -> Mux4/5, Retracted Leg Trajectory/7(dphi_apex)
  Alpha Target to Leg Length and Leg Angle/3(ddl) -> Mux4/3
  Alpha Target to Leg Length and Leg Angle/4(phi) -> Mux4/4, Retracted Leg Trajectory/6(phi_apex)
  Detect Fall Nonpositive/1 -> Retracted Leg Trajectory/1(start)
  Escape [1/0]/1 -> Signal During Escape/Enable, Detect Fall Nonpositive/1
  Retracted Leg Trajectory/5(dphi) -> Mux1/5
  Retracted Leg Trajectory/2(dl) -> Mux1/2
  Retracted Leg Trajectory/4(phi) -> Mux1/4
  Retracted Leg Trajectory/1(l) -> Mux1/1
  AlphaRef/1 -> Terminator5/1
  Sum1/1 -> Compare To Constant/1, Signal During Escape/1(time)
  Alpha Target Law l0 = 1.037112 m k = 23000 N/m target height = 1.137112 m target speed = 0.5 m/s m = 60.4120 kg g = 5.9004 m/s^2 E = 412.882588 J/1(AlphaRef(t) [rad]) -> Alpha Target to Leg Length and Leg Angle/1(alpha_v), AlphaRef/1
  Clock/1 -> Sum1/1, Retracted Leg Trajectory/2(t_system)
  Apex Time [s]/1 -> Sum1/2, Retracted Leg Trajectory/3(t_apex)
  Mux1/1 -> Switch/3
  Torso Pitch [rad rad/s]/1 -> Demux1/1

== system smm_with_grf_tilting_2d/Control/Behavior Control/Primary Leg Behavior/Running/Flight/Deadbeat Placement/Leg Trajectory Generator (Normal) ==
  Leg Length [m m/s] : Inport
  Leg Angle [rad rad/s] : Inport  Port=2
  Torso Pitch [rad rad/s] : Inport  Port=3
  Apex Time [s] : Inport  Port=4
  Escape [1/0] : Inport  Port=5
  Alpha Target Law l0 = 1.037112 m k = 8820 N/m target height = 1.057112 m target speed = 1.0 m/s m = 60.4120 kg g = 5.900428 m/s^2 E = 444.778054 J : Subsystem
  Alpha Target to Leg Length and Leg Angle : MATLAB Function  TreatAsAtomicUnit=on
  AlphaRef : Gain
  Avoid Virtual Leg Length Limits : MATLAB Function  TreatAsAtomicUnit=on
  Avoid Virtual Leg Length Limits1 : MATLAB Function  TreatAsAtomicUnit=on
  Clock : Clock
  Compare To Constant : simulink/Logic and Bit Operations/Compare To Constant  relop=>  const=0  OutDataTypeStr=boolean  ZeroCross=off
  Demux : Demux  Outputs=6
  Demux1 : Demux  Outputs=2
  Demux2 : Demux  Outputs=2
  Demux3 : Demux  Outputs=2
  Detect Fall Nonpositive : simulink/Logic and Bit Operations/Detect Fall Nonpositive  vinit=0  InputProcessing=Inherited  OutDataTypeStr=boolean
  Mux1 : Mux  Inputs=6
  Mux2 : Mux  Inputs=3
  Mux3 : Mux  Inputs=3
  Mux4 : Mux  Inputs=6
  Retracted Leg Trajectory : MATLAB Function  TreatAsAtomicUnit=on
  Sum1 : Sum  Inputs=|+-
  Switch : Switch  Criteria=u2 ~= 0
  Terminator5 : Terminator
  Leg Length Target [m m/s m/s^2] : Outport
  Leg Angle Target [rad rad/s rad/s^2] : Outport  Port=2
  wires:
  Retracted Leg Trajectory/3(ddl) -> Avoid Virtual Leg Length Limits1/3(ddl_leg_desired)
  Retracted Leg Trajectory/2(dl) -> Avoid Virtual Leg Length Limits1/2(dl_leg_desired)
  Retracted Leg Trajectory/1(l) -> Avoid Virtual Leg Length Limits1/1(l_leg_desired)
  Avoid Virtual Leg Length Limits1/3(ddl_leg_cmd) -> Mux1/3
  Avoid Virtual Leg Length Limits1/2(dl_leg_cmd) -> Mux1/2
  Avoid Virtual Leg Length Limits1/1(l_leg_cmd) -> Mux1/1
  Alpha Target to Leg Length and Leg Angle/3(ddl) -> Avoid Virtual Leg Length Limits/3(ddl_leg_desired)
  Alpha Target to Leg Length and Leg Angle/2(dl) -> Avoid Virtual Leg Length Limits/2(dl_leg_desired)
  Alpha Target to Leg Length and Leg Angle/1(l) -> Avoid Virtual Leg Length Limits/1(l_leg_desired)
  Escape [1/0]/1 -> Detect Fall Nonpositive/1
  Torso Pitch [rad rad/s]/1 -> Demux1/1
  Mux1/1 -> Switch/3
  Compare To Constant/1 -> Switch/2
  Apex Time [s]/1 -> Sum1/2, Retracted Leg Trajectory/3(t_apex)
  Clock/1 -> Sum1/1, Retracted Leg Trajectory/2(t_system)
  Alpha Target Law l0 = 1.037112 m k = 8820 N/m target height = 1.057112 m target speed = 1.0 m/s m = 60.4120 kg g = 5.900428 m/s^2 E = 444.778054 J/1(AlphaRef(t) [rad]) -> AlphaRef/1, Alpha Target to Leg Length and Leg Angle/1(alpha_v)
  Sum1/1 -> Alpha Target Law l0 = 1.037112 m k = 8820 N/m target height = 1.057112 m target speed = 1.0 m/s m = 60.4120 kg g = 5.900428 m/s^2 E = 444.778054 J/1(tFall [s]), Compare To Constant/1
  AlphaRef/1 -> Terminator5/1
  Retracted Leg Trajectory/4(phi) -> Mux1/4
  Retracted Leg Trajectory/5(dphi) -> Mux1/5
  Detect Fall Nonpositive/1 -> Retracted Leg Trajectory/1(start)
  Alpha Target to Leg Length and Leg Angle/4(phi) -> Mux4/4, Retracted Leg Trajectory/6(phi_apex)
  Avoid Virtual Leg Length Limits/3(ddl_leg_cmd) -> Mux4/3
  Alpha Target to Leg Length and Leg Angle/5(dphi) -> Mux4/5, Retracted Leg Trajectory/7(dphi_apex)
  Alpha Target to Leg Length and Leg Angle/6(ddphi) -> Mux4/6
  Avoid Virtual Leg Length Limits/2(dl_leg_cmd) -> Mux4/2, Retracted Leg Trajectory/5(dl_apex)
  Avoid Virtual Leg Length Limits/1(l_leg_cmd) -> Mux4/1, Retracted Leg Trajectory/4(l_apex)
  Switch/1 -> Demux/1
  Mux2/1 -> Leg Length Target [m m/s m/s^2]/1
  Mux3/1 -> Leg Angle Target [rad rad/s rad/s^2]/1
  Demux/6 -> Mux3/3
  Demux/5 -> Mux3/2
  Demux/4 -> Mux3/1
  Demux/3 -> Mux2/3
  Demux/2 -> Mux2/2
  Demux/1 -> Mux2/1
  Demux1/1 -> Alpha Target to Leg Length and Leg Angle/4(theta)
  Demux1/2 -> Alpha Target to Leg Length and Leg Angle/5(dtheta)
  Mux4/1 -> Switch/1
  Alpha Target Law l0 = 1.037112 m k = 8820 N/m target height = 1.057112 m target speed = 1.0 m/s m = 60.4120 kg g = 5.900428 m/s^2 E = 444.778054 J/3(ddAlphaRef(t) [rad/s^2]) -> Alpha Target to Leg Length and Leg Angle/3(ddalpha_v)
  Alpha Target Law l0 = 1.037112 m k = 8820 N/m target height = 1.057112 m target speed = 1.0 m/s m = 60.4120 kg g = 5.900428 m/s^2 E = 444.778054 J/2(dAlphaRef(t) [rad/s]) -> Alpha Target to Leg Length and Leg Angle/2(dalpha_v)
  Retracted Leg Trajectory/6(ddphi) -> Mux1/6
  Demux2/1 -> Retracted Leg Trajectory/8(l_measured)
  Demux2/2 -> Retracted Leg Trajectory/9(dl_measured)
  Demux3/1 -> Retracted Leg Trajectory/10(phi_measured)
  Demux3/2 -> Retracted Leg Trajectory/11(dphi_measured)
  Leg Angle [rad rad/s]/1 -> Demux3/1
  Leg Length [m m/s]/1 -> Demux2/1

== system smm_with_grf_tilting_2d/Control/Behavior Control/Primary Leg Behavior/Running/Flight/Hold Values/Subsystem ==
  in : Inport
  Enable : EnablePort
  out : Outport  InitialOutput=[0 0 l0_leg l0_leg]
  wires:
  in/1 -> out/1

== system smm_with_grf_tilting_2d/Control/Behavior Control/Primary Leg Behavior/Running/Stance/Calculate Spring Rest Length/Hold Initial ==
  in : Inport
  Trigger : TriggerPort  ShowOutputPort=on  PortDimensions=1
  Subsystem : Subsystem
  out : Outport
  wires:
  Trigger/1 -> Subsystem/Enable
  Subsystem/1(out) -> out/1
  in/1 -> Subsystem/1(in)

== system smm_with_grf_tilting_2d/Control/Behavior Control/Primary Leg Behavior/Running/Stance/Inverse Dynamics Virtual Spring/Leg Force-Torque Distribution ==
  Front Spring Torque [Nm] : Inport
  Back Spring Torque [Nm] : Inport  Port=2
  w [m] : Inport  Port=3
  Divide : Product  Inputs=*/
  Sum2 : Sum  Inputs=+|+
  Sum5 : Sum  Inputs=+|-
  Leg Force [N] : Outport
  Leg Torque [Nm] : Outport  Port=2
  wires:
  Sum2/1 -> Leg Torque [Nm]/1
  Back Spring Torque [Nm]/1 -> Sum5/2, Sum2/2
  Sum5/1 -> Divide/1
  w [m]/1 -> Divide/2
  Front Spring Torque [Nm]/1 -> Sum5/1, Sum2/1
  Divide/1 -> Leg Force [N]/1

== system smm_with_grf_tilting_2d/Control/Behavior Control/Primary Leg Behavior/Running/Flight/Deadbeat Placement/Back//Front Motor PD/Friction Compensation ==
  Right/Left [1/0] : Inport
  Commanded Velocity [rad/s] [back front] : Inport  Port=2
  Product : Product
  Sign : Signum
  Sum1 : Sum
  Switch : Switch  Criteria=u2 ~= 0
  Switch1 : Switch  Criteria=u2 ~= 0
  coulomb_friction_left : Constant  Value=sea_coulomb_friction(3:4)
  coulomb_friction_right : Constant  Value=sea_coulomb_friction(1:2)
  offset_friction_left : Constant  Value=sea_offset_friction(3:4)
  offset_friction_right : Constant  Value=sea_offset_friction(1:2)
  Friction Compensation [Nm] : Outport
  wires:
  Commanded Velocity [rad/s] [back front]/1 -> Sign/1
  Switch/1 -> Sum1/2
  Sum1/1 -> Friction Compensation [Nm]/1
  Product/1 -> Sum1/1
  Right/Left [1/0]/1 -> Switch1/2, Switch/2
  offset_friction_right/1 -> Switch/1
  offset_friction_left/1 -> Switch/3
  coulomb_friction_right/1 -> Switch1/1
  coulomb_friction_left/1 -> Switch1/3
  Switch1/1 -> Product/2
  Sign/1 -> Product/1

== system smm_with_grf_tilting_2d/Control/Behavior Control/Primary Leg Behavior/Running/Flight/Deadbeat Placement/Leg Trajectory Generator (Level Ground)/Alpha Target Law l0 = 1.037112 m k = 23000 N//m target height = 1.137112 m target speed = 0.5 m//s m = 60.4120 kg g = 5.9004 m//s^2 E = 412.882588 J ==
  note: Angle of Attack Control Law From Poincare Map Method
  tFall [s] : Inport
  Alpha Target Polynomials : Subsystem
  AlphaRef1 : Constant  Value=[(90+20)*pi/180 0 0]
  Compare To Constant1 : simulink/Logic and Bit Operations/Compare To Constant  relop=<  const=0.19512514  OutDataTypeStr=boolean  ZeroCross=off
  Demux : Demux  Outputs=3
  Ignore Negatives : Fcn  Expr=(u >= 0)*u
  Mux : Mux  Inputs=3
  Switch : Switch  Criteria=u2 ~= 0
  AlphaRef(t) [rad] : Outport
  dAlphaRef(t) [rad/s] : Outport  Port=2
  ddAlphaRef(t) [rad/s^2] : Outport  Port=3
  wires:
  Ignore Negatives/1 -> Alpha Target Polynomials/1(tFall)
  Mux/1 -> Switch/1
  Alpha Target Polynomials/1(AlphaRef(t)) -> Mux/1
  Alpha Target Polynomials/3(ddAlphaRef(t)) -> Mux/3
  Alpha Target Polynomials/2(dAlphaRef(t)) -> Mux/2
  Compare To Constant1/1 -> Switch/2
  tFall [s]/1 -> Compare To Constant1/1, Ignore Negatives/1
  Switch/1 -> Demux/1
  Demux/1 -> AlphaRef(t) [rad]/1
  Demux/2 -> dAlphaRef(t) [rad/s]/1
  Demux/3 -> ddAlphaRef(t) [rad/s^2]/1
  AlphaRef1/1 -> Switch/3

== system smm_with_grf_tilting_2d/Control/Behavior Control/Primary Leg Behavior/Running/Flight/Deadbeat Placement/Leg Trajectory Generator (Level Ground)/Signal During Escape ==
  time : Inport
  Enable : EnablePort
  time to apex [s] : Outport
  wires:
  time/1 -> time to apex [s]/1

== system smm_with_grf_tilting_2d/Control/Behavior Control/Primary Leg Behavior/Running/Flight/Deadbeat Placement/Leg Trajectory Generator (Normal)/Alpha Target Law l0 = 1.037112 m k = 8820 N//m target height = 1.057112 m target speed = 1.0 m//s m = 60.4120 kg g = 5.900428 m//s^2 E = 444.778054 J ==
  note: Angle of Attack Control Law From Poincare Map Method
  tFall [s] : Inport
  Alpha Target Polynomials : Subsystem
  AlphaRef1 : Constant  Value=[(90+20)*pi/180 0 0]
  Compare To Constant1 : simulink/Logic and Bit Operations/Compare To Constant  relop=<  const=0.33124891  OutDataTypeStr=boolean  ZeroCross=off
  Demux : Demux  Outputs=3
  Ignore Negatives : Fcn  Expr=(u >= 0)*u
  Mux : Mux  Inputs=3
  Switch : Switch  Criteria=u2 ~= 0
  AlphaRef(t) [rad] : Outport
  dAlphaRef(t) [rad/s] : Outport  Port=2
  ddAlphaRef(t) [rad/s^2] : Outport  Port=3
  wires:
  Alpha Target Polynomials/1(AlphaRef(t)) -> Mux/1
  AlphaRef1/1 -> Switch/3
  Demux/3 -> ddAlphaRef(t) [rad/s^2]/1
  Demux/2 -> dAlphaRef(t) [rad/s]/1
  Demux/1 -> AlphaRef(t) [rad]/1
  Switch/1 -> Demux/1
  tFall [s]/1 -> Ignore Negatives/1, Compare To Constant1/1
  Compare To Constant1/1 -> Switch/2
  Alpha Target Polynomials/2(dAlphaRef(t)) -> Mux/2
  Alpha Target Polynomials/3(ddAlphaRef(t)) -> Mux/3
  Mux/1 -> Switch/1
  Ignore Negatives/1 -> Alpha Target Polynomials/1(tFall)

== system smm_with_grf_tilting_2d/Control/Behavior Control/Primary Leg Behavior/Running/Stance/Calculate Spring Rest Length/Hold Initial/Subsystem ==
  in : Inport
  Enable : EnablePort
  out : Outport  InitialOutput=[l0_virtual]
  wires:
  in/1 -> out/1

== system smm_with_grf_tilting_2d/Control/Behavior Control/Primary Leg Behavior/Running/Flight/Deadbeat Placement/Leg Trajectory Generator (Level Ground)/Alpha Target Law l0 = 1.037112 m k = 23000 N//m target height = 1.137112 m target speed = 0.5 m//s m = 60.4120 kg g = 5.9004 m//s^2 E = 412.882588 J/Alpha Target Polynomials ==
  tFall : Inport
  AlphaRef(t) Control Law : Fcn  Expr=1.0339*u^3 + 6.848*u^2 + 3.5731*u + alpha_apex
  acceleration of AlphaRef(t) Control Law : Fcn  Expr=2*3*1.0339*u + 2*6.848
  velocity of AlphaRef(t) Control Law : Fcn  Expr=3*1.0339*u^2 + 2*6.848*u + 3.5731
  AlphaRef(t) : Outport  OutputWhenDisabled=reset  InitialOutput=0
      settings: AttributesFormatString=When disabled: %<OutputWhenDisabled>\nDisabled Output: %<InitialOutput>
  dAlphaRef(t) : Outport  Port=2  OutputWhenDisabled=reset  InitialOutput=0
      settings: AttributesFormatString=When disbaled: %<OutputWhenDisabled>\nDisabled output: %<InitialOutput>
  ddAlphaRef(t) : Outport  Port=3  OutputWhenDisabled=reset  InitialOutput=0
      settings: AttributesFormatString=When disabled: %<OutputWhenDisabled>\nDisabled output: %<InitialOutput>
  wires:
  tFall/1 -> AlphaRef(t) Control Law/1, velocity of AlphaRef(t) Control Law/1, acceleration of AlphaRef(t) Control Law/1
  AlphaRef(t) Control Law/1 -> AlphaRef(t)/1
  velocity of AlphaRef(t) Control Law/1 -> dAlphaRef(t)/1
  acceleration of AlphaRef(t) Control Law/1 -> ddAlphaRef(t)/1

== system smm_with_grf_tilting_2d/Control/Behavior Control/Primary Leg Behavior/Running/Flight/Deadbeat Placement/Leg Trajectory Generator (Normal)/Alpha Target Law l0 = 1.037112 m k = 8820 N//m target height = 1.057112 m target speed = 1.0 m//s m = 60.4120 kg g = 5.900428 m//s^2 E = 444.778054 J/Alpha Target Polynomials ==
  tFall : Inport
  AlphaRef(t) Control Law : Fcn  Expr=12.835*u^3 - 2.9736*u^2 + 1.9343*u + alpha_apex
  acceleration of AlphaRef(t) Control Law : Fcn  Expr=2*3*12.835*u - 2*2.9736
  velocity of AlphaRef(t) Control Law : Fcn  Expr=3*12.835*u^2 - 2*2.9736*u + 1.9343
  AlphaRef(t) : Outport  OutputWhenDisabled=reset  InitialOutput=0
      settings: AttributesFormatString=When disabled: %<OutputWhenDisabled>\nDisabled Output: %<InitialOutput>
  dAlphaRef(t) : Outport  Port=2  OutputWhenDisabled=reset  InitialOutput=0
      settings: AttributesFormatString=When disbaled: %<OutputWhenDisabled>\nDisabled output: %<InitialOutput>
  ddAlphaRef(t) : Outport  Port=3  OutputWhenDisabled=reset  InitialOutput=0
      settings: AttributesFormatString=When disabled: %<OutputWhenDisabled>\nDisabled output: %<InitialOutput>
  wires:
  acceleration of AlphaRef(t) Control Law/1 -> ddAlphaRef(t)/1
  velocity of AlphaRef(t) Control Law/1 -> dAlphaRef(t)/1
  AlphaRef(t) Control Law/1 -> AlphaRef(t)/1
  tFall/1 -> acceleration of AlphaRef(t) Control Law/1, velocity of AlphaRef(t) Control Law/1, AlphaRef(t) Control Law/1

== stateflow chart smm_with_grf_tilting_2d/Control/Behavior Control/Primary Leg Behavior/State Machine ==
  state TouchDown
  state LockedContact
  state Unloading
  state Takeoff
  state Flight
  (junction 91) -> TouchDown
  TouchDown -> (junction 130) [order 2] : [vertical_grf < contact_threshold]
  (junction 93) -> (junction 91)
  (junction 130) -> (junction 128)
  TouchDown -> LockedContact [order 1] : [vertical_grf > loaded_threshold]
  (junction 115) -> LockedContact
  (junction 118) -> (junction 115)
  LockedContact -> Unloading : [leg_velocity >= 0 && previous_leg_velocity < 0]
  Unloading -> LockedContact [order 2] : [vertical_grf > loaded_threshold && leg_velocity < 0]
  (junction 122) -> (junction 118)
  Unloading -> Takeoff [order 1] : [vertical_grf < contact_threshold || leg_length > max_leg_length]
  Takeoff -> Flight : after(t_flight,sec)
  (default) -> Flight
  Flight -> (junction 93) : [vertical_grf > contact_threshold]
  (junction 128) -> Flight
  data: leg_length input; leg_velocity input; previous_leg_velocity input; vertical_grf input; t_flight parameter; max_leg_length parameter; contact_threshold parameter; loaded_threshold parameter; TouchDown output boolean; LockedContact output boolean; Unloading output boolean; Takeoff output boolean; Flight output boolean
